simulink model "TST_AFS_VDDrftComp"  (R2016b)
settings: Solver=FixedStepDiscrete  StartTime=0.0  StopTime=simTime  FixedStep=sampleTime  RelTol=1e-3
values from neighbouring files (symbols this model uses):
  testCase = 1    [initTST_AFS_VDDrftComp_001.m]
libraries: simulink x8, UnitTest_Lib x6
settings Model: Creator=zhengjinyan  LastModifiedBy=zhengjinyan
settings DebuggingCC: SignalRangeChecking=error

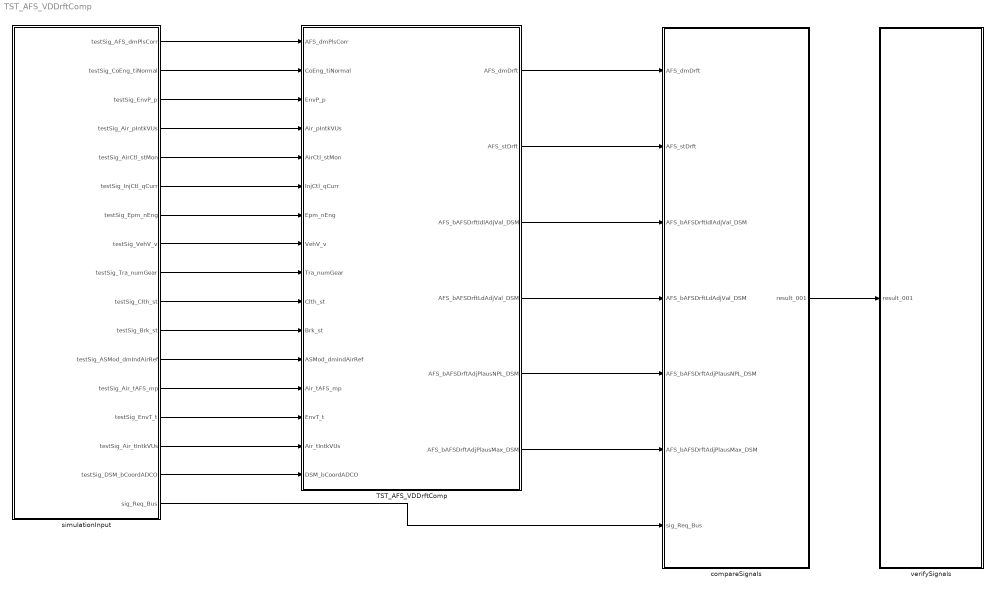
== system TST_AFS_VDDrftComp ==
  TST_AFS_VDDrftComp : Subsystem
  compareSignals : Subsystem
  simulationInput : Subsystem
  verifySignals : Subsystem
  wires:
  simulationInput/1(testSig_AFS_dmPlsCorr) -> TST_AFS_VDDrftComp/1(AFS_dmPlsCorr)
  simulationInput/2(testSig_CoEng_tiNormal) -> TST_AFS_VDDrftComp/2(CoEng_tiNormal)
  simulationInput/3(testSig_EnvP_p) -> TST_AFS_VDDrftComp/3(EnvP_p)
  simulationInput/4(testSig_Air_pIntkVUs) -> TST_AFS_VDDrftComp/4(Air_pIntkVUs)
  simulationInput/5(testSig_AirCtl_stMon) -> TST_AFS_VDDrftComp/5(AirCtl_stMon)
  simulationInput/6(testSig_InjCtl_qCurr) -> TST_AFS_VDDrftComp/6(InjCtl_qCurr)
  simulationInput/7(testSig_Epm_nEng) -> TST_AFS_VDDrftComp/7(Epm_nEng)
  simulationInput/8(testSig_VehV_v) -> TST_AFS_VDDrftComp/8(VehV_v)
  simulationInput/9(testSig_Tra_numGear) -> TST_AFS_VDDrftComp/9(Tra_numGear)
  simulationInput/10(testSig_Clth_st) -> TST_AFS_VDDrftComp/10(Clth_st)
  simulationInput/11(testSig_Brk_st) -> TST_AFS_VDDrftComp/11(Brk_st)
  simulationInput/12(testSig_ASMod_dmIndAirRef) -> TST_AFS_VDDrftComp/12(ASMod_dmIndAirRef)
  simulationInput/13(testSig_Air_tAFS_mp) -> TST_AFS_VDDrftComp/13(Air_tAFS_mp)
  simulationInput/14(testSig_EnvT_t) -> TST_AFS_VDDrftComp/14(EnvT_t)
  simulationInput/15(testSig_Air_tIntkVUs) -> TST_AFS_VDDrftComp/15(Air_tIntkVUs)
  simulationInput/16(testSig_DSM_bCoordADCO) -> TST_AFS_VDDrftComp/16(DSM_bCoordADCO)
  TST_AFS_VDDrftComp/1(AFS_dmDrft) -> compareSignals/1(AFS_dmDrft)
  TST_AFS_VDDrftComp/2(AFS_stDrft) -> compareSignals/2(AFS_stDrft)
  TST_AFS_VDDrftComp/3(AFS_bAFSDrftIdlAdjVal_DSM) -> compareSignals/3(AFS_bAFSDrftIdlAdjVal_DSM)
  TST_AFS_VDDrftComp/4(AFS_bAFSDrftLdAdjVal_DSM) -> compareSignals/4(AFS_bAFSDrftLdAdjVal_DSM)
  TST_AFS_VDDrftComp/5(AFS_bAFSDrftAdjPlausNPL_DSM) -> compareSignals/5(AFS_bAFSDrftAdjPlausNPL_DSM)
  TST_AFS_VDDrftComp/6(AFS_bAFSDrftAdjPlausMax_DSM) -> compareSignals/6(AFS_bAFSDrftAdjPlausMax_DSM)
  simulationInput/17(sig_Req_Bus) -> compareSignals/7(sig_Req_Bus)
  compareSignals/1(result_001) -> verifySignals/1(result_001)

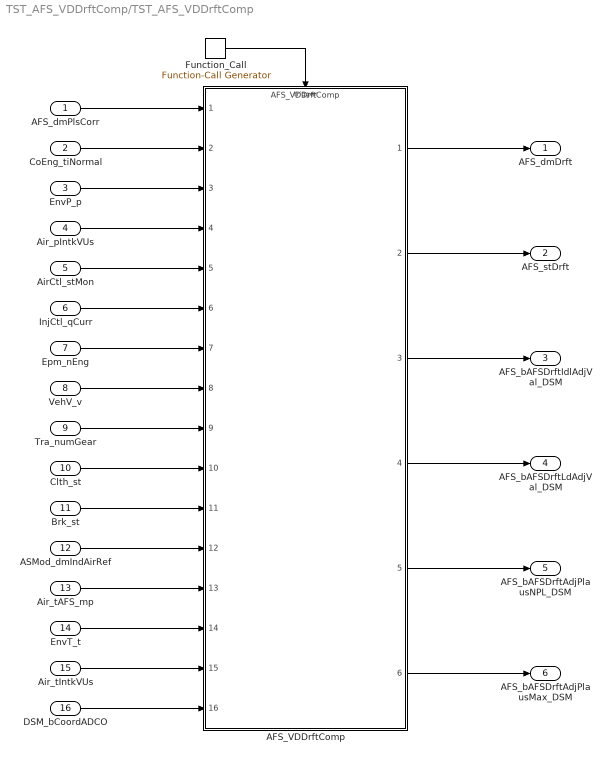
== system TST_AFS_VDDrftComp/TST_AFS_VDDrftComp ==
  AFS_dmPlsCorr : Inport
  CoEng_tiNormal : Inport  Port=2
  EnvP_p : Inport  Port=3
  Air_pIntkVUs : Inport  Port=4
  AirCtl_stMon : Inport  Port=5
  InjCtl_qCurr : Inport  Port=6
  Epm_nEng : Inport  Port=7
  VehV_v : Inport  Port=8
  Tra_numGear : Inport  Port=9
  Clth_st : Inport  Port=10
  Brk_st : Inport  Port=11
  ASMod_dmIndAirRef : Inport  Port=12
  Air_tAFS_mp : Inport  Port=13
  EnvT_t : Inport  Port=14
  Air_tIntkVUs : Inport  Port=15
  DSM_bCoordADCO : Inport  Port=16
  AFS_VDDrftComp : ModelReference  ModelNameDialog=AFS_VDDrftComp  SimulationMode=Normal  ModelReferenceVersion=1.50  TriggerPortName=function  TriggerPortTriggerType=function-call  TriggerPortStatesWhenEnabling=held
  Function_Call : simulink/Ports & Subsystems/Function-Call Generator  sample_time=sampleTime  numberOfIterations=1
  AFS_dmDrft : Outport
  AFS_stDrft : Outport  Port=2
  AFS_bAFSDrftIdlAdjVal_DSM : Outport  Port=3
  AFS_bAFSDrftLdAdjVal_DSM : Outport  Port=4
  AFS_bAFSDrftAdjPlausNPL_DSM : Outport  Port=5
  AFS_bAFSDrftAdjPlausMax_DSM : Outport  Port=6
  wires:
  Function_Call/1 -> AFS_VDDrftComp/Trigger
  AFS_dmPlsCorr/1 -> AFS_VDDrftComp/1
  CoEng_tiNormal/1 -> AFS_VDDrftComp/2
  EnvP_p/1 -> AFS_VDDrftComp/3
  Air_pIntkVUs/1 -> AFS_VDDrftComp/4
  AirCtl_stMon/1 -> AFS_VDDrftComp/5
  InjCtl_qCurr/1 -> AFS_VDDrftComp/6
  Epm_nEng/1 -> AFS_VDDrftComp/7
  VehV_v/1 -> AFS_VDDrftComp/8
  Tra_numGear/1 -> AFS_VDDrftComp/9
  Clth_st/1 -> AFS_VDDrftComp/10
  Brk_st/1 -> AFS_VDDrftComp/11
  ASMod_dmIndAirRef/1 -> AFS_VDDrftComp/12
  Air_tAFS_mp/1 -> AFS_VDDrftComp/13
  EnvT_t/1 -> AFS_VDDrftComp/14
  Air_tIntkVUs/1 -> AFS_VDDrftComp/15
  DSM_bCoordADCO/1 -> AFS_VDDrftComp/16
  AFS_VDDrftComp/1 -> AFS_dmDrft/1
  AFS_VDDrftComp/2 -> AFS_stDrft/1
  AFS_VDDrftComp/3 -> AFS_bAFSDrftIdlAdjVal_DSM/1
  AFS_VDDrftComp/4 -> AFS_bAFSDrftLdAdjVal_DSM/1
  AFS_VDDrftComp/5 -> AFS_bAFSDrftAdjPlausNPL_DSM/1
  AFS_VDDrftComp/6 -> AFS_bAFSDrftAdjPlausMax_DSM/1

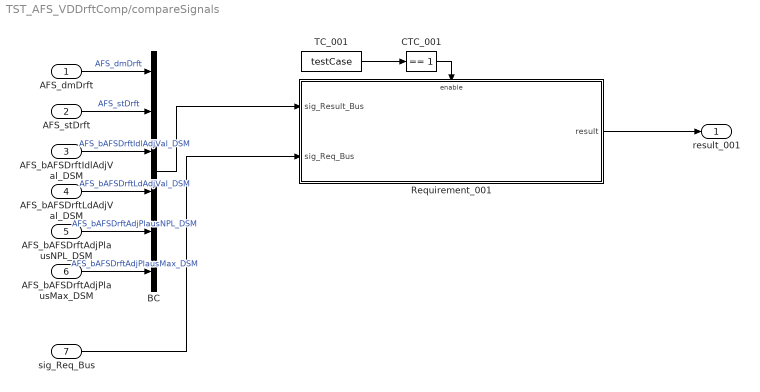
== system TST_AFS_VDDrftComp/compareSignals ==
  AFS_dmDrft : Inport
  AFS_stDrft : Inport  Port=2
  AFS_bAFSDrftIdlAdjVal_DSM : Inport  Port=3
  AFS_bAFSDrftLdAdjVal_DSM : Inport  Port=4
  AFS_bAFSDrftAdjPlausNPL_DSM : Inport  Port=5
  AFS_bAFSDrftAdjPlausMax_DSM : Inport  Port=6
  sig_Req_Bus : Inport  Port=7
  BC : BusCreator  Inputs=6
  CTC_001 : simulink/Logic and Bit Operations/Compare To Constant  relop===  const=1  OutDataTypeStr=boolean
  Requirement_001 : Subsystem
  TC_001 : Constant  Value=testCase
  result_001 : Outport
  wires:
  AFS_dmDrft/1 -> BC/1  "AFS_dmDrft"
  AFS_stDrft/1 -> BC/2  "AFS_stDrft"
  AFS_bAFSDrftIdlAdjVal_DSM/1 -> BC/3  "AFS_bAFSDrftIdlAdjVal_DSM"
  AFS_bAFSDrftLdAdjVal_DSM/1 -> BC/4  "AFS_bAFSDrftLdAdjVal_DSM"
  AFS_bAFSDrftAdjPlausNPL_DSM/1 -> BC/5  "AFS_bAFSDrftAdjPlausNPL_DSM"
  AFS_bAFSDrftAdjPlausMax_DSM/1 -> BC/6  "AFS_bAFSDrftAdjPlausMax_DSM"
  TC_001/1 -> CTC_001/1
  CTC_001/1 -> Requirement_001/Enable
  sig_Req_Bus/1 -> Requirement_001/2(sig_Req_Bus)
  BC/1 -> Requirement_001/1(sig_Result_Bus)
  Requirement_001/1(result) -> result_001/1

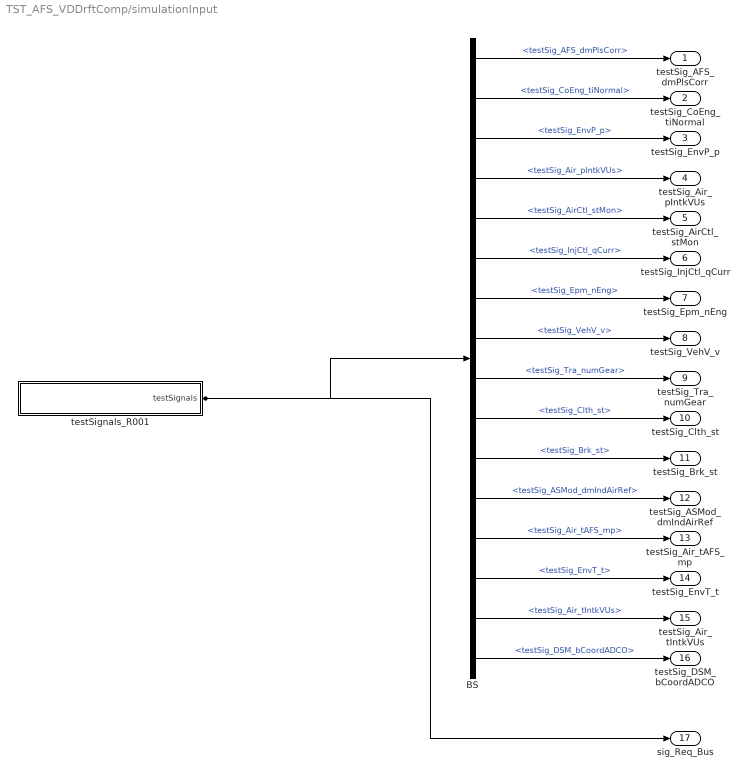
== system TST_AFS_VDDrftComp/simulationInput ==
  BS : BusSelector  OutputSignals=testSig_AFS_dmPlsCorr,testSig_CoEng_tiNormal,testSig_EnvP_p,testSig_Air_pIntkVUs,testSig_AirCtl_stMon,testSig_InjCtl_qCurr,testSig_Epm_nEng,testSig_VehV_v,testSig_Tra_numGear,testSig_Clth_st,testSig_Brk_st,testSig_ASMod_dmIndAirRef,testSig_Air_tAFS_mp,testSig_EnvT_t,testSig_Air_tIntkVUs,testSig_DSM_bCoordADCO
  testSignals_R001 : Subsystem
  testSig_AFS_dmPlsCorr : Outport
  testSig_CoEng_tiNormal : Outport  Port=2
  testSig_EnvP_p : Outport  Port=3
  testSig_Air_pIntkVUs : Outport  Port=4
  testSig_AirCtl_stMon : Outport  Port=5
  testSig_InjCtl_qCurr : Outport  Port=6
  testSig_Epm_nEng : Outport  Port=7
  testSig_VehV_v : Outport  Port=8
  testSig_Tra_numGear : Outport  Port=9
  testSig_Clth_st : Outport  Port=10
  testSig_Brk_st : Outport  Port=11
  testSig_ASMod_dmIndAirRef : Outport  Port=12
  testSig_Air_tAFS_mp : Outport  Port=13
  testSig_EnvT_t : Outport  Port=14
  testSig_Air_tIntkVUs : Outport  Port=15
  testSig_DSM_bCoordADCO : Outport  Port=16
  sig_Req_Bus : Outport  Port=17
  wires:
  BS/1 -> testSig_AFS_dmPlsCorr/1  "<testSig_AFS_dmPlsCorr>"
  BS/2 -> testSig_CoEng_tiNormal/1  "<testSig_CoEng_tiNormal>"
  BS/3 -> testSig_EnvP_p/1  "<testSig_EnvP_p>"
  BS/4 -> testSig_Air_pIntkVUs/1  "<testSig_Air_pIntkVUs>"
  BS/5 -> testSig_AirCtl_stMon/1  "<testSig_AirCtl_stMon>"
  BS/6 -> testSig_InjCtl_qCurr/1  "<testSig_InjCtl_qCurr>"
  BS/7 -> testSig_Epm_nEng/1  "<testSig_Epm_nEng>"
  BS/8 -> testSig_VehV_v/1  "<testSig_VehV_v>"
  BS/9 -> testSig_Tra_numGear/1  "<testSig_Tra_numGear>"
  BS/10 -> testSig_Clth_st/1  "<testSig_Clth_st>"
  BS/11 -> testSig_Brk_st/1  "<testSig_Brk_st>"
  BS/12 -> testSig_ASMod_dmIndAirRef/1  "<testSig_ASMod_dmIndAirRef>"
  BS/13 -> testSig_Air_tAFS_mp/1  "<testSig_Air_tAFS_mp>"
  BS/14 -> testSig_EnvT_t/1  "<testSig_EnvT_t>"
  BS/15 -> testSig_Air_tIntkVUs/1  "<testSig_Air_tIntkVUs>"
  BS/16 -> testSig_DSM_bCoordADCO/1  "<testSig_DSM_bCoordADCO>"
  testSignals_R001/1(testSignals) -> BS/1, sig_Req_Bus/1

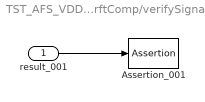
== system TST_AFS_VDDrftComp/verifySignals ==
  result_001 : Inport
  Assertion_001 : Assertion  Enabled=off
  wires:
  result_001/1 -> Assertion_001/1

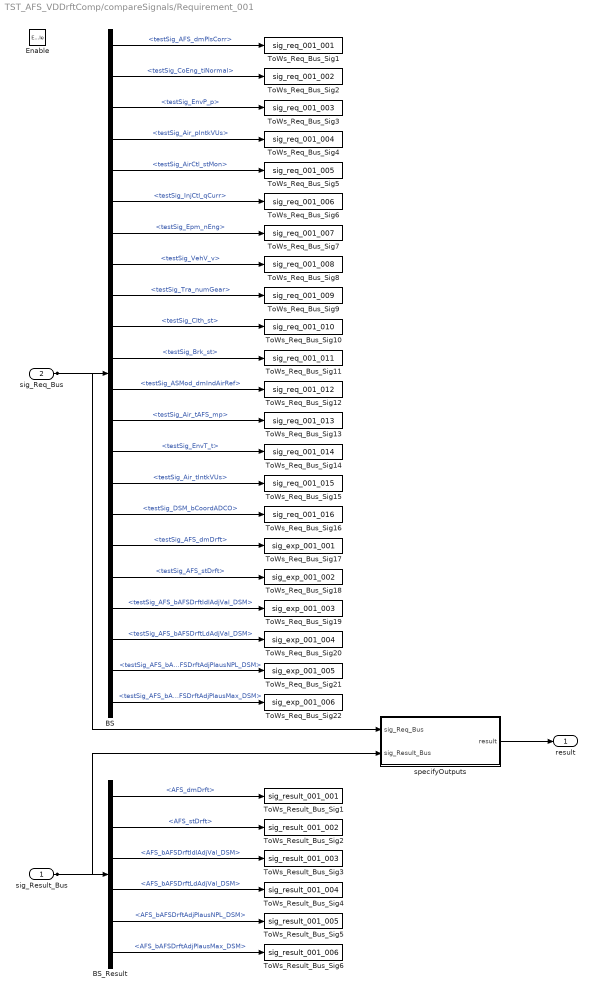
== system TST_AFS_VDDrftComp/compareSignals/Requirement_001 ==
  sig_Result_Bus : Inport
  sig_Req_Bus : Inport  Port=2
  Enable : EnablePort
  BS : BusSelector  OutputSignals=testSig_AFS_dmPlsCorr,testSig_CoEng_tiNormal,testSig_EnvP_p,testSig_Air_pIntkVUs,testSig_AirCtl_stMon,testSig_InjCtl_qCurr,testSig_Epm_nEng,testSig_VehV_v,testSig_Tra_numGear,testSig_Clth_st,testSig_Brk_st,testSig_ASMod_dmIndAirRef,testSig_Air_tAFS_mp,testSig_EnvT_t,testSig_Air_tIntkVUs,testSig_DSM_bCoordADCO,testSig_AFS_dmDrft,testSig_AFS_stDrft,testSig_AFS_bAFSDrftIdlAdjVal_DSM,testSig_AFS_bAFSDrftLdAdjVal_DSM,testSig_AFS_bAFSDrftAdjPlausNPL_DSM,testSig_AFS_bAFSDrftAdjPlausMax_DSM
  BS_Result : BusSelector  OutputSignals=AFS_dmDrft,AFS_stDrft,AFS_bAFSDrftIdlAdjVal_DSM,AFS_bAFSDrftLdAdjVal_DSM,AFS_bAFSDrftAdjPlausNPL_DSM,AFS_bAFSDrftAdjPlausMax_DSM
  ToWs_Req_Bus_Sig1 : ToWorkspace  VariableName=sig_req_001_001  SaveFormat=Structure With Time
  ToWs_Req_Bus_Sig10 : ToWorkspace  VariableName=sig_req_001_010  SaveFormat=Structure With Time
  ToWs_Req_Bus_Sig11 : ToWorkspace  VariableName=sig_req_001_011  SaveFormat=Structure With Time
  ToWs_Req_Bus_Sig12 : ToWorkspace  VariableName=sig_req_001_012  SaveFormat=Structure With Time
  ToWs_Req_Bus_Sig13 : ToWorkspace  VariableName=sig_req_001_013  SaveFormat=Structure With Time
  ToWs_Req_Bus_Sig14 : ToWorkspace  VariableName=sig_req_001_014  SaveFormat=Structure With Time
  ToWs_Req_Bus_Sig15 : ToWorkspace  VariableName=sig_req_001_015  SaveFormat=Structure With Time
  ToWs_Req_Bus_Sig16 : ToWorkspace  VariableName=sig_req_001_016  SaveFormat=Structure With Time
  ToWs_Req_Bus_Sig17 : ToWorkspace  VariableName=sig_exp_001_001  SaveFormat=Structure With Time
  ToWs_Req_Bus_Sig18 : ToWorkspace  VariableName=sig_exp_001_002  SaveFormat=Structure With Time
  ToWs_Req_Bus_Sig19 : ToWorkspace  VariableName=sig_exp_001_003  SaveFormat=Structure With Time
  ToWs_Req_Bus_Sig2 : ToWorkspace  VariableName=sig_req_001_002  SaveFormat=Structure With Time
  ToWs_Req_Bus_Sig20 : ToWorkspace  VariableName=sig_exp_001_004  SaveFormat=Structure With Time
  ToWs_Req_Bus_Sig21 : ToWorkspace  VariableName=sig_exp_001_005  SaveFormat=Structure With Time
  ToWs_Req_Bus_Sig22 : ToWorkspace  VariableName=sig_exp_001_006  SaveFormat=Structure With Time
  ToWs_Req_Bus_Sig3 : ToWorkspace  VariableName=sig_req_001_003  SaveFormat=Structure With Time
  ToWs_Req_Bus_Sig4 : ToWorkspace  VariableName=sig_req_001_004  SaveFormat=Structure With Time
  ToWs_Req_Bus_Sig5 : ToWorkspace  VariableName=sig_req_001_005  SaveFormat=Structure With Time
  ToWs_Req_Bus_Sig6 : ToWorkspace  VariableName=sig_req_001_006  SaveFormat=Structure With Time
  ToWs_Req_Bus_Sig7 : ToWorkspace  VariableName=sig_req_001_007  SaveFormat=Structure With Time
  ToWs_Req_Bus_Sig8 : ToWorkspace  VariableName=sig_req_001_008  SaveFormat=Structure With Time
  ToWs_Req_Bus_Sig9 : ToWorkspace  VariableName=sig_req_001_009  SaveFormat=Structure With Time
  ToWs_Result_Bus_Sig1 : ToWorkspace  VariableName=sig_result_001_001  SaveFormat=Structure With Time
  ToWs_Result_Bus_Sig2 : ToWorkspace  VariableName=sig_result_001_002  SaveFormat=Structure With Time
  ToWs_Result_Bus_Sig3 : ToWorkspace  VariableName=sig_result_001_003  SaveFormat=Structure With Time
  ToWs_Result_Bus_Sig4 : ToWorkspace  VariableName=sig_result_001_004  SaveFormat=Structure With Time
  ToWs_Result_Bus_Sig5 : ToWorkspace  VariableName=sig_result_001_005  SaveFormat=Structure With Time
  ToWs_Result_Bus_Sig6 : ToWorkspace  VariableName=sig_result_001_006  SaveFormat=Structure With Time
  specifyOutputs : Subsystem
  result : Outport
  wires:
  sig_Req_Bus/1 -> BS/1, specifyOutputs/1(sig_Req_Bus)
  BS/1 -> ToWs_Req_Bus_Sig1/1  "<testSig_AFS_dmPlsCorr>"
  BS/2 -> ToWs_Req_Bus_Sig2/1  "<testSig_CoEng_tiNormal>"
  BS/3 -> ToWs_Req_Bus_Sig3/1  "<testSig_EnvP_p>"
  BS/4 -> ToWs_Req_Bus_Sig4/1  "<testSig_Air_pIntkVUs>"
  BS/5 -> ToWs_Req_Bus_Sig5/1  "<testSig_AirCtl_stMon>"
  BS/6 -> ToWs_Req_Bus_Sig6/1  "<testSig_InjCtl_qCurr>"
  BS/7 -> ToWs_Req_Bus_Sig7/1  "<testSig_Epm_nEng>"
  BS/8 -> ToWs_Req_Bus_Sig8/1  "<testSig_VehV_v>"
  BS/9 -> ToWs_Req_Bus_Sig9/1  "<testSig_Tra_numGear>"
  BS/10 -> ToWs_Req_Bus_Sig10/1  "<testSig_Clth_st>"
  BS/11 -> ToWs_Req_Bus_Sig11/1  "<testSig_Brk_st>"
  BS/12 -> ToWs_Req_Bus_Sig12/1  "<testSig_ASMod_dmIndAirRef>"
  BS/13 -> ToWs_Req_Bus_Sig13/1  "<testSig_Air_tAFS_mp>"
  BS/14 -> ToWs_Req_Bus_Sig14/1  "<testSig_EnvT_t>"
  BS/15 -> ToWs_Req_Bus_Sig15/1  "<testSig_Air_tIntkVUs>"
  BS/16 -> ToWs_Req_Bus_Sig16/1  "<testSig_DSM_bCoordADCO>"
  BS/17 -> ToWs_Req_Bus_Sig17/1  "<testSig_AFS_dmDrft>"
  BS/18 -> ToWs_Req_Bus_Sig18/1  "<testSig_AFS_stDrft>"
  BS/19 -> ToWs_Req_Bus_Sig19/1  "<testSig_AFS_bAFSDrftIdlAdjVal_DSM>"
  BS/20 -> ToWs_Req_Bus_Sig20/1  "<testSig_AFS_bAFSDrftLdAdjVal_DSM>"
  BS/21 -> ToWs_Req_Bus_Sig21/1  "<testSig_AFS_bAFSDrftAdjPlausNPL_DSM>"
  BS/22 -> ToWs_Req_Bus_Sig22/1  "<testSig_AFS_bAFSDrftAdjPlausMax_DSM>"
  sig_Result_Bus/1 -> BS_Result/1, specifyOutputs/2(sig_Result_Bus)
  BS_Result/1 -> ToWs_Result_Bus_Sig1/1  "<AFS_dmDrft>"
  BS_Result/2 -> ToWs_Result_Bus_Sig2/1  "<AFS_stDrft>"
  BS_Result/3 -> ToWs_Result_Bus_Sig3/1  "<AFS_bAFSDrftIdlAdjVal_DSM>"
  BS_Result/4 -> ToWs_Result_Bus_Sig4/1  "<AFS_bAFSDrftLdAdjVal_DSM>"
  BS_Result/5 -> ToWs_Result_Bus_Sig5/1  "<AFS_bAFSDrftAdjPlausNPL_DSM>"
  BS_Result/6 -> ToWs_Result_Bus_Sig6/1  "<AFS_bAFSDrftAdjPlausMax_DSM>"
  specifyOutputs/1(result) -> result/1

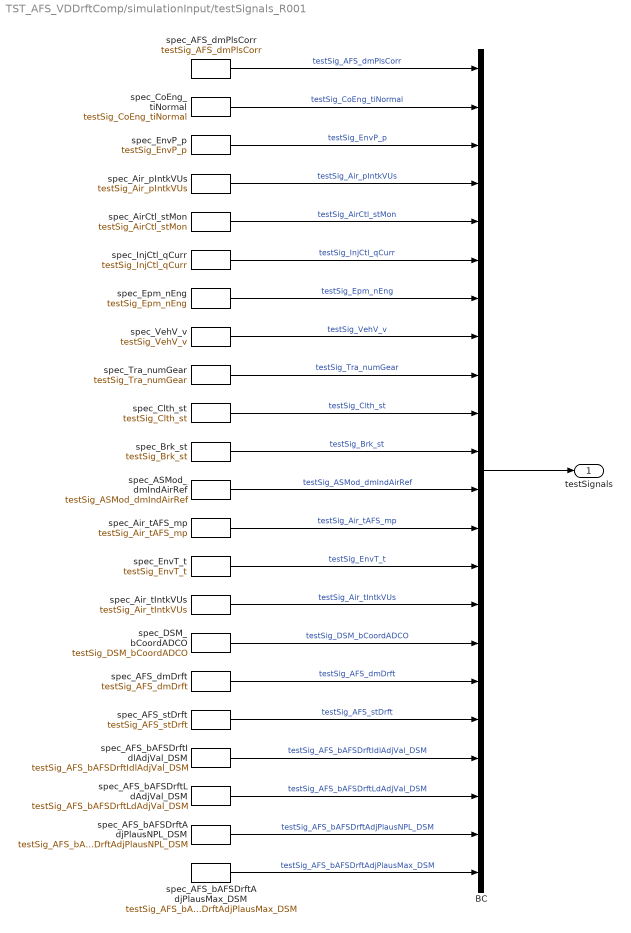
== system TST_AFS_VDDrftComp/simulationInput/testSignals_R001 ==
  BC : BusCreator  Inputs=22
  spec_AFS_bAFSDrftAdjPlausMax_DSM : FromWorkspace  VariableName=testSig_AFS_bAFSDrftAdjPlausMax_DSM  Interpolate=off  OutputAfterFinalValue=Holding final value
  spec_AFS_bAFSDrftAdjPlausNPL_DSM : FromWorkspace  VariableName=testSig_AFS_bAFSDrftAdjPlausNPL_DSM  Interpolate=off  OutputAfterFinalValue=Holding final value
  spec_AFS_bAFSDrftIdlAdjVal_DSM : FromWorkspace  VariableName=testSig_AFS_bAFSDrftIdlAdjVal_DSM  Interpolate=off  OutputAfterFinalValue=Holding final value
  spec_AFS_bAFSDrftLdAdjVal_DSM : FromWorkspace  VariableName=testSig_AFS_bAFSDrftLdAdjVal_DSM  Interpolate=off  OutputAfterFinalValue=Holding final value
  spec_AFS_dmDrft : FromWorkspace  VariableName=testSig_AFS_dmDrft  Interpolate=off  OutputAfterFinalValue=Holding final value
  spec_AFS_dmPlsCorr : FromWorkspace  VariableName=testSig_AFS_dmPlsCorr  Interpolate=off  OutputAfterFinalValue=Holding final value
  spec_AFS_stDrft : FromWorkspace  VariableName=testSig_AFS_stDrft  Interpolate=off  OutputAfterFinalValue=Holding final value
  spec_ASMod_dmIndAirRef : FromWorkspace  VariableName=testSig_ASMod_dmIndAirRef  Interpolate=off  OutputAfterFinalValue=Holding final value
  spec_AirCtl_stMon : FromWorkspace  VariableName=testSig_AirCtl_stMon  Interpolate=off  OutputAfterFinalValue=Holding final value
  spec_Air_pIntkVUs : FromWorkspace  VariableName=testSig_Air_pIntkVUs  Interpolate=off  OutputAfterFinalValue=Holding final value
  spec_Air_tAFS_mp : FromWorkspace  VariableName=testSig_Air_tAFS_mp  Interpolate=off  OutputAfterFinalValue=Holding final value
  spec_Air_tIntkVUs : FromWorkspace  VariableName=testSig_Air_tIntkVUs  Interpolate=off  OutputAfterFinalValue=Holding final value
  spec_Brk_st : FromWorkspace  VariableName=testSig_Brk_st  Interpolate=off  OutputAfterFinalValue=Holding final value
  spec_Clth_st : FromWorkspace  VariableName=testSig_Clth_st  Interpolate=off  OutputAfterFinalValue=Holding final value
  spec_CoEng_tiNormal : FromWorkspace  VariableName=testSig_CoEng_tiNormal  Interpolate=off  OutputAfterFinalValue=Holding final value
  spec_DSM_bCoordADCO : FromWorkspace  VariableName=testSig_DSM_bCoordADCO  Interpolate=off  OutputAfterFinalValue=Holding final value
  spec_EnvP_p : FromWorkspace  VariableName=testSig_EnvP_p  Interpolate=off  OutputAfterFinalValue=Holding final value
  spec_EnvT_t : FromWorkspace  VariableName=testSig_EnvT_t  Interpolate=off  OutputAfterFinalValue=Holding final value
  spec_Epm_nEng : FromWorkspace  VariableName=testSig_Epm_nEng  Interpolate=off  OutputAfterFinalValue=Holding final value
  spec_InjCtl_qCurr : FromWorkspace  VariableName=testSig_InjCtl_qCurr  Interpolate=off  OutputAfterFinalValue=Holding final value
  spec_Tra_numGear : FromWorkspace  VariableName=testSig_Tra_numGear  Interpolate=off  OutputAfterFinalValue=Holding final value
  spec_VehV_v : FromWorkspace  VariableName=testSig_VehV_v  Interpolate=off  OutputAfterFinalValue=Holding final value
  testSignals : Outport
  wires:
  BC/1 -> testSignals/1
  spec_AFS_dmPlsCorr/1 -> BC/1  "testSig_AFS_dmPlsCorr"
  spec_CoEng_tiNormal/1 -> BC/2  "testSig_CoEng_tiNormal"
  spec_EnvP_p/1 -> BC/3  "testSig_EnvP_p"
  spec_Air_pIntkVUs/1 -> BC/4  "testSig_Air_pIntkVUs"
  spec_AirCtl_stMon/1 -> BC/5  "testSig_AirCtl_stMon"
  spec_InjCtl_qCurr/1 -> BC/6  "testSig_InjCtl_qCurr"
  spec_Epm_nEng/1 -> BC/7  "testSig_Epm_nEng"
  spec_VehV_v/1 -> BC/8  "testSig_VehV_v"
  spec_Tra_numGear/1 -> BC/9  "testSig_Tra_numGear"
  spec_Clth_st/1 -> BC/10  "testSig_Clth_st"
  spec_Brk_st/1 -> BC/11  "testSig_Brk_st"
  spec_ASMod_dmIndAirRef/1 -> BC/12  "testSig_ASMod_dmIndAirRef"
  spec_Air_tAFS_mp/1 -> BC/13  "testSig_Air_tAFS_mp"
  spec_EnvT_t/1 -> BC/14  "testSig_EnvT_t"
  spec_Air_tIntkVUs/1 -> BC/15  "testSig_Air_tIntkVUs"
  spec_DSM_bCoordADCO/1 -> BC/16  "testSig_DSM_bCoordADCO"
  spec_AFS_dmDrft/1 -> BC/17  "testSig_AFS_dmDrft"
  spec_AFS_stDrft/1 -> BC/18  "testSig_AFS_stDrft"
  spec_AFS_bAFSDrftIdlAdjVal_DSM/1 -> BC/19  "testSig_AFS_bAFSDrftIdlAdjVal_DSM"
  spec_AFS_bAFSDrftLdAdjVal_DSM/1 -> BC/20  "testSig_AFS_bAFSDrftLdAdjVal_DSM"
  spec_AFS_bAFSDrftAdjPlausNPL_DSM/1 -> BC/21  "testSig_AFS_bAFSDrftAdjPlausNPL_DSM"
  spec_AFS_bAFSDrftAdjPlausMax_DSM/1 -> BC/22  "testSig_AFS_bAFSDrftAdjPlausMax_DSM"

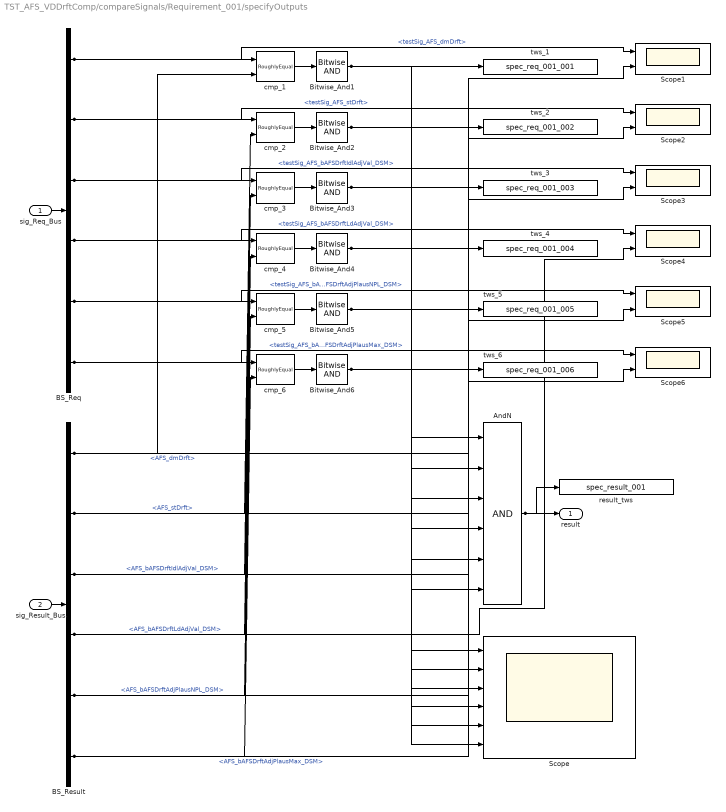
== system TST_AFS_VDDrftComp/compareSignals/Requirement_001/specifyOutputs ==
  sig_Req_Bus : Inport
  sig_Result_Bus : Inport  Port=2
  AndN : Logic  Inputs=6
  BS_Req : BusSelector  OutputSignals=testSig_AFS_dmDrft,testSig_AFS_stDrft,testSig_AFS_bAFSDrftIdlAdjVal_DSM,testSig_AFS_bAFSDrftLdAdjVal_DSM,testSig_AFS_bAFSDrftAdjPlausNPL_DSM,testSig_AFS_bAFSDrftAdjPlausMax_DSM
  BS_Result : BusSelector  OutputSignals=AFS_dmDrft,AFS_stDrft,AFS_bAFSDrftIdlAdjVal_DSM,AFS_bAFSDrftLdAdjVal_DSM,AFS_bAFSDrftAdjPlausNPL_DSM,AFS_bAFSDrftAdjPlausMax_DSM
  Bitwise_And{1..6} (6 alike) : simulink/Logic and Bit Operations/Bitwise Operator  logicop=AND  UseBitMask=off  BitMask=bin2dec('11011001')  BitMaskRealWorld=Stored Integer
  Scope : Scope  NumInputPorts=6
  Scope{1..6} (6 alike) : Scope  NumInputPorts=2
  cmp_{1..6} (6 alike) : UnitTest_Lib/RoughlyEqual  slope=0.1
  result_tws : ToWorkspace  VariableName=spec_result_001
  tws_1 : ToWorkspace  VariableName=spec_req_001_001
  tws_2 : ToWorkspace  VariableName=spec_req_001_002
  tws_3 : ToWorkspace  VariableName=spec_req_001_003
  tws_4 : ToWorkspace  VariableName=spec_req_001_004
  tws_5 : ToWorkspace  VariableName=spec_req_001_005
  tws_6 : ToWorkspace  VariableName=spec_req_001_006
  result : Outport
  wires:
  sig_Req_Bus/1 -> BS_Req/1
  sig_Result_Bus/1 -> BS_Result/1
  AndN/1 -> result/1, result_tws/1
  BS_Req/1 -> cmp_1/1, Scope1/1  "<testSig_AFS_dmDrft>"
  BS_Result/1 -> cmp_1/2, Scope1/2  "<AFS_dmDrft>"
  cmp_1/1 -> Bitwise_And1/1
  Bitwise_And1/1 -> tws_1/1, AndN/1, Scope/1
  BS_Req/2 -> cmp_2/1, Scope2/1  "<testSig_AFS_stDrft>"
  BS_Result/2 -> cmp_2/2, Scope2/2  "<AFS_stDrft>"
  cmp_2/1 -> Bitwise_And2/1
  Bitwise_And2/1 -> tws_2/1, AndN/2, Scope/2
  BS_Req/3 -> cmp_3/1, Scope3/1  "<testSig_AFS_bAFSDrftIdlAdjVal_DSM>"
  BS_Result/3 -> cmp_3/2, Scope3/2  "<AFS_bAFSDrftIdlAdjVal_DSM>"
  cmp_3/1 -> Bitwise_And3/1
  Bitwise_And3/1 -> tws_3/1, AndN/3, Scope/3
  BS_Req/4 -> cmp_4/1, Scope4/1  "<testSig_AFS_bAFSDrftLdAdjVal_DSM>"
  BS_Result/4 -> cmp_4/2, Scope4/2  "<AFS_bAFSDrftLdAdjVal_DSM>"
  cmp_4/1 -> Bitwise_And4/1
  Bitwise_And4/1 -> tws_4/1, AndN/4, Scope/4
  BS_Req/5 -> cmp_5/1, Scope5/1  "<testSig_AFS_bAFSDrftAdjPlausNPL_DSM>"
  BS_Result/5 -> cmp_5/2, Scope5/2  "<AFS_bAFSDrftAdjPlausNPL_DSM>"
  cmp_5/1 -> Bitwise_And5/1
  Bitwise_And5/1 -> tws_5/1, AndN/5, Scope/5
  BS_Req/6 -> cmp_6/1, Scope6/1  "<testSig_AFS_bAFSDrftAdjPlausMax_DSM>"
  BS_Result/6 -> cmp_6/2, Scope6/2  "<AFS_bAFSDrftAdjPlausMax_DSM>"
  cmp_6/1 -> Bitwise_And6/1
  Bitwise_And6/1 -> tws_6/1, AndN/6, Scope/6
